simulink model "pcm_line"  (R2018b)
settings: Solver=VariableStepAuto  StartTime=0.0  StopTime=168  RelTol=1e-3
libraries: dsparch4 x6, commsrccod2 x2, commblkcod2 x2, commutil2 x2, commchan3 x1, dspsrcs4 x1, commsink2 x1
settings Model: Creator=lance  LastModifiedBy=lance

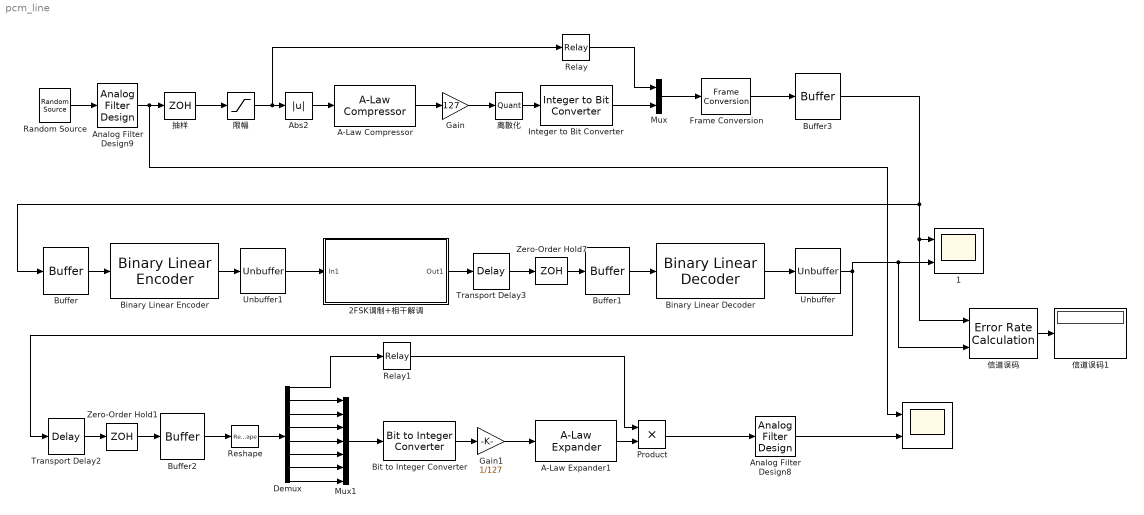
== system pcm_line ==
  " " : Scope  NumInputPorts=2
  " 1" : Scope  NumInputPorts=2
  "2FSK调制+相干解调 " : Subsystem
  A-Law Compressor : commsrccod2/A-Law Compressor  A=87.6  V=1
      settings: SourceProductName=Communications System Toolbox  SourceProductBaseCode=CM
  A-Law Expander1 : commsrccod2/A-Law Expander  A=87.6  V=1
      settings: SourceProductName=Communications System Toolbox  SourceProductBaseCode=CM
  Abs2 : Abs
  Analog Filter Design8 : dsparch4/Analog Filter Design  method=Butterworth  filttype=Lowpass  N=8  Wlo=0.15*2*pi  Whi=210*2*pi  Rp=2  Rs=40
  Analog Filter Design9 : dsparch4/Analog Filter Design  method=Butterworth  filttype=Lowpass  N=8  Wlo=2*pi*0.1  Whi=103*2*pi  Rp=2  Rs=40
  Binary Linear Decoder : commblkcod2/Binary Linear Decoder  G=[[1 1 0; 1 1 1;1 0 1] eye(3)]  trt=0
      settings: SourceProductName=Communications System Toolbox  SourceProductBaseCode=CM
  Binary Linear Encoder : commblkcod2/Binary Linear Encoder  G=[[1 1 0; 1 1 1; 1 0 1] eye(3)]
      settings: SourceProductName=Communications System Toolbox  SourceProductBaseCode=CM
  Bit to Integer Converter : commutil2/Bit to Integer Converter  nbits=7  bitOrder=MSB first  signedOutputValues=Unsigned  outDtype=Inherit via internal rule  outDtypeSigned=Inherit via internal rule
  Buffer : Buffer  N=3  OutputFrames=off
  Buffer1 : Buffer  N=6  OutputFrames=off
  Buffer2 : Buffer  N=8  OutputFrames=off
  Buffer3 : Buffer  N=1  OutputFrames=off
  Demux : Demux  Outputs=8
  Frame Conversion : FrameConversion
  Gain : Gain  Gain=127
  Gain1 : Gain  Gain=1/127
  Integer to Bit Converter : commutil2/Integer to Bit Converter  nbits=7  signedInputValues=Unsigned  bitOrder=MSB first  outDtype=Inherit via internal rule
  Mux : Mux  Inputs=2
  Mux1 : Mux  Inputs=7
  Product : Product  RndMeth=Zero
  Random Source : dspsrcs4/Random Source  SrcType=Uniform  NormMethod=Ziggurat  CltLength=12  MinVal=-1  MaxVal=1  MeanVal=0  VarVal=1  RepMode=Repeatable  rawSeed=56  IsInherit=off  SampMode=Discrete  SampTime=0.001  SampFrame=1  DataType=Double  OutComplex=Real  OutputFrames=off
  Relay : Relay
  Relay1 : Relay  OffOutputValue=-1
  Reshape : Reshape
  Transport Delay2 : TransportDelay  DelayTime=2.8
  Transport Delay3 : TransportDelay  DelayTime=0.8
  Unbuffer : Unbuffer
  Unbuffer1 : Unbuffer
  Zero-Order Hold1 : ZeroOrderHold  SampleTime=0.4
  Zero-Order Hold7 : ZeroOrderHold  SampleTime=0.2
  信道误码 : commsink2/Error Rate Calculation  N=9  st_delay=0  cp_mode=Entire frame  subframe=[]  PMode=Port  WsName=ErrorVec  RsMode2=off  stop=off  numErr=100  maxBits=1e6
  "信道误码1 " : Display
  抽样 : ZeroOrderHold  SampleTime=3.2
  离散化 : Quantizer  QuantizationInterval=1
  限幅 : Saturate  UpperLimit=1  LowerLimit=-1
  wires:
  Buffer/1 -> Binary Linear Encoder/1
  Binary Linear Encoder/1 -> Unbuffer1/1
  Unbuffer1/1 -> "2FSK调制+相干解调 "/1(In1)
  Binary Linear Decoder/1 -> Unbuffer/1
  Zero-Order Hold7/1 -> Buffer1/1
  Buffer1/1 -> Binary Linear Decoder/1
  Transport Delay3/1 -> Zero-Order Hold7/1
  "2FSK调制+相干解调 "/1(Out1) -> Transport Delay3/1
  Zero-Order Hold1/1 -> Buffer2/1
  Gain1/1 -> A-Law Expander1/1
  Buffer2/1 -> Reshape/1
  Demux/6 -> Mux1/5
  Transport Delay2/1 -> Zero-Order Hold1/1
  Demux/2 -> Mux1/1
  Unbuffer/1 -> 信道误码/2, " 1"/2, Transport Delay2/1
  Bit to Integer Converter/1 -> Gain1/1
  A-Law Expander1/1 -> Product/2
  Demux/5 -> Mux1/4
  Demux/4 -> Mux1/3
  Demux/3 -> Mux1/2
  Relay1/1 -> Product/1
  Mux1/1 -> Bit to Integer Converter/1
  Reshape/1 -> Demux/1
  Demux/7 -> Mux1/6
  Demux/8 -> Mux1/7
  Demux/1 -> Relay1/1
  Product/1 -> Analog Filter Design8/1
  Random Source/1 -> Analog Filter Design9/1
  抽样/1 -> 限幅/1
  离散化/1 -> Integer to Bit Converter/1
  A-Law Compressor/1 -> Gain/1
  Relay/1 -> Mux/1
  Mux/1 -> Frame Conversion/1
  Gain/1 -> 离散化/1
  Abs2/1 -> A-Law Compressor/1
  Analog Filter Design9/1 -> " "/1, 抽样/1
  Integer to Bit Converter/1 -> Mux/2
  限幅/1 -> Relay/1, Abs2/1
  Frame Conversion/1 -> Buffer3/1
  Buffer3/1 -> Buffer/1, 信道误码/1, " 1"/1
  Analog Filter Design8/1 -> " "/2
  信道误码/1 -> "信道误码1 "/1

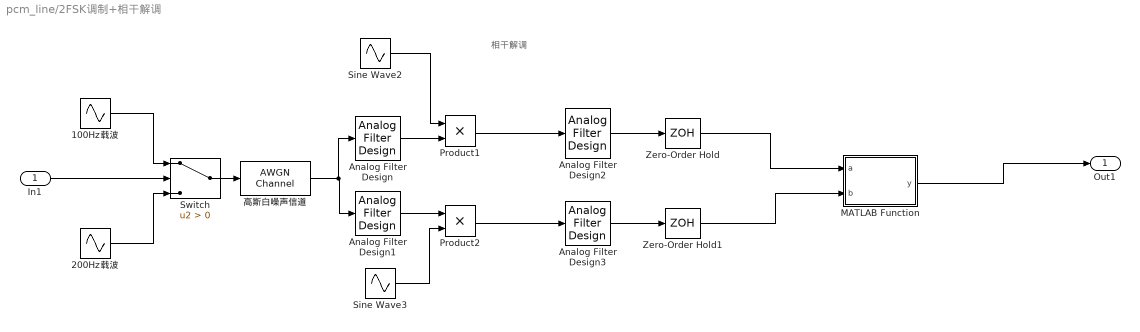
== system pcm_line/2FSK调制+相干解调  ==
  note: 相干解调
  In1 : Inport
  100Hz载波 : Sin  Frequency=100*2*pi  SampleTime=0.0001
  200Hz载波 : Sin  Frequency=200*2*pi  SampleTime=0.0001
  Analog Filter Design : dsparch4/Analog Filter Design  method=Butterworth  filttype=Bandpass  N=8  Wlo=90*2*pi  Whi=110*2*pi  Rp=2  Rs=40
  Analog Filter Design1 : dsparch4/Analog Filter Design  method=Butterworth  filttype=Bandpass  N=8  Wlo=190*2*pi  Whi=210*2*pi  Rp=2  Rs=40
  Analog Filter Design2 : dsparch4/Analog Filter Design  method=Butterworth  filttype=Lowpass  N=8  Wlo=10*pi  Whi=103*2*pi  Rp=2  Rs=40
  Analog Filter Design3 : dsparch4/Analog Filter Design  method=Butterworth  filttype=Lowpass  N=8  Wlo=10*pi  Whi=103*2*pi  Rp=2  Rs=40
  MATLAB Function : MATLAB Function  TreatAsAtomicUnit=on
  Product1 : Product
  Product2 : Product
  Sine Wave2 : Sin  Frequency=100*2*pi  SampleTime=0.0001
  Sine Wave3 : Sin  Frequency=200*2*pi  SampleTime=0.0001
  Switch : Switch  Criteria=u2 > Threshold
  Zero-Order Hold : ZeroOrderHold  SampleTime=0.2
  Zero-Order Hold1 : ZeroOrderHold  SampleTime=0.2
  "高斯白噪声信道 " : commchan3/AWGN Channel  InputProcessing=Columns as channels (frame based)  seed=67  noiseMode="Signal to noise ratio  (SNR)"  EbNodB=1  EsNodB=10  SNRdB=-20  bitsPerSym=1  Ps=1  Tsym=1  variance=1
  Out1 : Outport
  wires:
  In1/1 -> Switch/2
  "高斯白噪声信道 "/1 -> Analog Filter Design1/1, Analog Filter Design/1
  Analog Filter Design3/1 -> Zero-Order Hold1/1
  100Hz载波/1 -> Switch/1
  Sine Wave3/1 -> Product2/2
  Switch/1 -> "高斯白噪声信道 "/1
  Product1/1 -> Analog Filter Design2/1
  Analog Filter Design/1 -> Product1/2
  200Hz载波/1 -> Switch/3
  Zero-Order Hold1/1 -> MATLAB Function/2(b)
  Sine Wave2/1 -> Product1/1
  Analog Filter Design2/1 -> Zero-Order Hold/1
  Zero-Order Hold/1 -> MATLAB Function/1(a)
  Analog Filter Design1/1 -> Product2/1
  Product2/1 -> Analog Filter Design3/1
  MATLAB Function/1(y) -> Out1/1

== matlab function pcm_line/2FSK调制+相干解调 /MATLAB Function ==
  data: a input; y output; b input
function y = fcn(a, b)
if(a>b)
    y=1;
else
    y=0;
end
